simulink model "ex02_led_pwm_sample"  (R2016a)
settings: Solver=FixedStepDiscrete  StartTime=0.0  StopTime=10  RelTol=1e-3
libraries: embdlinuxlib x1
settings Model: ModifiedByFormat=The MathWorks Inc.  Creator=The MathWorks, Inc.  LastModifiedBy=The MathWorks Inc.
settings SolverCC: PositivePriorityOrder=on
settings DataIOCC: LimitDataPoints=on  SaveFormat=Array
settings OptimizationCC: OptimizeModelRefInitCode=on  LifeSpan=1  MaxStackSize=64
settings DebuggingCC: UnderspecifiedInitializationDetection=Classic  MergeDetectMultiDrivingBlocksExec=none  SolverPrmCheckMsg=warning  AllowSymbolicDim=off
settings HardwareCC: ProdBitPerPointer=32  ProdLargestAtomicInteger=Long  ProdLargestAtomicFloat=Double  ProdWordSize=32  ProdHWDeviceType=ARM Compatible->ARM Cortex  UseEmbeddedCoderFeatures=off  UseSimulinkCoderFeatures=off
settings ModelReferenceCC: PropagateSignalLabelsOutOfModel=off
settings RTWCC: SystemTargetFile=ert.tlc  HardwareBoard=Raspberry Pi  TemplateMakefile=ert_default_tmf  Toolchain=GNU GCC Raspberry Pi
settings CodeAppCC: IgnoreCustomStorageClasses=off
settings ERTTargetCC: SupportNonInlinedSFcns=on  ConvertIfToSwitch=off  SuppressUnreachableDefaultCases=off
settings ConfigComp: CovModelRefEnable=Off  CovSFcnEnable=off

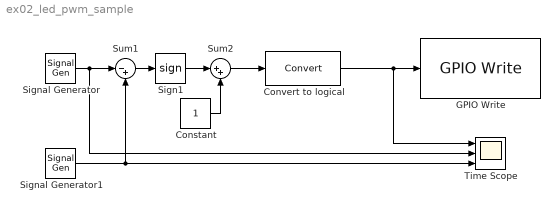
== system ex02_led_pwm_sample ==
  Constant : Constant  SampleTime=0.0001
  Convert to logical : DataTypeConversion
  GPIO Write : embdlinuxlib/GPIO Write  board=Pi 3 Model B  gpio=14  direction=Output  blockPlatform=Raspberry Pi
  Sign1 : Signum
  Signal Generator : SignalGenerator  Amplitude=1.1
  Signal Generator1 : SignalGenerator  WaveForm=sawtooth  Frequency=1000
  Sum1 : Sum  Inputs=|-+
  Sum2 : Sum  Inputs=|++
  Time Scope : Scope  NumInputPorts=3
  wires:
  Signal Generator/1 -> Time Scope/2, Sum1/1
  Signal Generator1/1 -> Time Scope/3, Sum1/2
  Sum1/1 -> Sign1/1
  Sign1/1 -> Sum2/1
  Sum2/1 -> Convert to logical/1
  Constant/1 -> Sum2/2
  Convert to logical/1 -> Time Scope/1, GPIO Write/1
